simulink model "Model_Rover"  (R2024a)
settings: Solver=VariableStepAuto  StartTime=0.0  StopTime=10.0  RelTol=1e-3
values from neighbouring files (symbols this model uses):
  sp = [0, 0]    [main.m]
  zp = [5, 5]    [main.m]
settings Model: Creator=thiagothielecke  LastModifiedBy=thiagothielecke

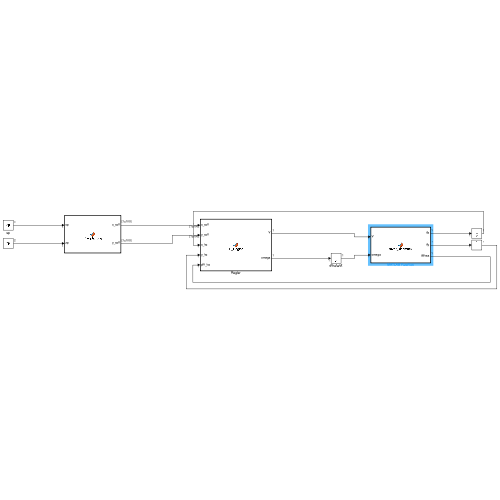
[thumbnail: Simulink's stored preview of the top-level diagram]
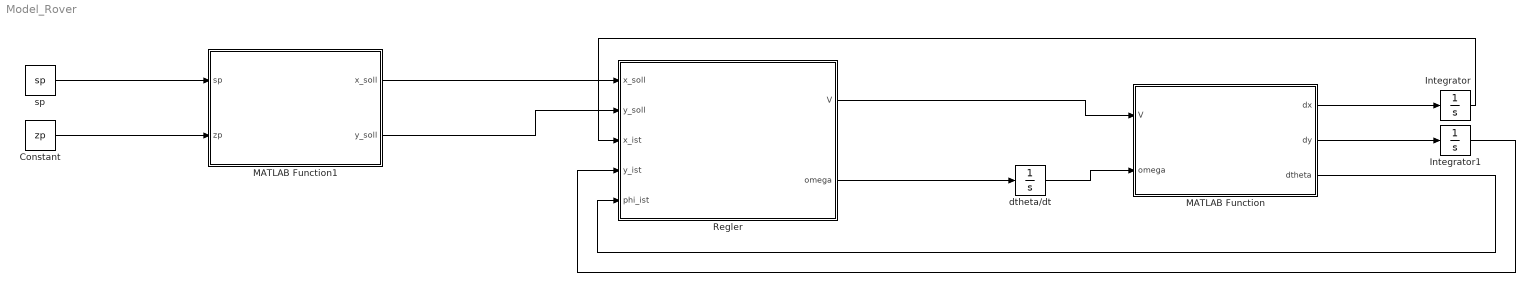
== system Model_Rover ==
  Constant : Constant  Value=zp
  Integrator : Integrator
  Integrator1 : Integrator
  MATLAB Function : MATLAB Function  TreatAsAtomicUnit=on
  MATLAB Function1 : MATLAB Function  TreatAsAtomicUnit=on
  Regler : MATLAB Function  TreatAsAtomicUnit=on
  dtheta/dt : Integrator
  sp : Constant  Value=sp
  wires:
  Regler/1(V) -> MATLAB Function/1(V)
  Regler/2(omega) -> dtheta/dt/1
  dtheta/dt/1 -> MATLAB Function/2(omega)
  MATLAB Function/2(dy) -> Integrator1/1
  MATLAB Function/1(dx) -> Integrator/1
  MATLAB Function/3(dtheta) -> Regler/5(phi_ist)
  Integrator1/1 -> Regler/4(y_ist)
  sp/1 -> MATLAB Function1/1(sp)
  Constant/1 -> MATLAB Function1/2(zp)
  MATLAB Function1/1(x_soll) -> Regler/1(x_soll)
  MATLAB Function1/2(y_soll) -> Regler/2(y_soll)
  Integrator/1 -> Regler/3(x_ist)

== matlab function Model_Rover/Regler ==
  data: x_soll input; V output; y_soll input; x_ist input; y_ist input; phi_ist input; omega output
function [V, omega] = P_Regler(x_soll, y_soll, x_ist, y_ist, phi_ist)

    % Parameter
    Kp_pos = 0.5;      % Verstärkung für Position
    Kp_phi = 0.5;      % Verstärkung für Richtung
    tol_dist = 0.01;   % Toleranz für Position
    tol_angle = 0.01;  % Toleranz für Winkel

    % Positionsfehler (Höhen- und Breitenunterschied)
    fehler_x = x_soll - x_ist;
    fehler_y = y_soll - y_ist;

    % Entfernung und Zielwinkel berechnen
    entfernung = sqrt(fehler_x^2 + fehler_y^2);
    winkel_zum_ziel = atan2(fehler_y, fehler_x);

    %Calculate the angle difference / error
    fehler_phi = winkel_zum_ziel - phi_ist;
    % Winkelabweichung normieren [pi, -pi]
    fehler_phi = atan2(sin(fehler_phi), cos(fehler_phi));

    % Standardwerte: Anhalten
    V = 0.0;
    omega = 0.0;

    if entfernung > tol_dist
        if abs(fehler_phi) > tol_angle
            % Nur rotieren
            omega = Kp_phi * fehler_phi;
            V = 0.0;
        else
            % Nur vorwärts bewegen
            V = Kp_pos * entfernung;
            omega = 0.0;
        end
    end

end

== matlab function Model_Rover/MATLAB Function ==
  data: dx output; V input; dy output; omega input; dtheta output
%% Berechnung der Rover-Kinematik
function [dx, dy, dtheta] = rover_kinematik(V, omega)

%% Eingaben:
%   V     - Vorwärtsgeschwindigkeit [m/s]
%   omega - Winkelgeschwindigkeit [rad/s]
%   theta - momentane Ausrichtung [rad]

%% Ausgaben:
%   dx    - Änderung der x-Position [m/s]
%   dy    - Änderung der y-Position [m/s]
%   dtheta- Änderung des Winkels [rad/s]

dx     = V * cos(theta);
dy     = V * sin(theta);
dtheta = omega;

%% hier Erweiterung der Rover Kinematik mit 4 Rädern

end

== matlab function Model_Rover/MATLAB Function1 ==
  data: sp input; x_soll output; zp input; y_soll output
function[x_soll, y_soll]= Pfadplanung(sp,zp)

%Eingabe
%sp- Startpunkt als Vektor
%zp-Zielpunkt als Vektor

%Anzahl Zwischenpunkte
N = 100;

%Gerade Linie von Start - Zielpunkt
x_soll = linspace(sp(1), zp(1), N);
y_soll = linspace(sp(2), zp(2), N);
end
